simulink model "Model"  (R2024b)
settings: Solver=VariableStepAuto  StartTime=0.0  StopTime=10.0  RelTol=1e-3
libraries: simulink x5
settings Model: Creator=ethansilver  LastModifiedBy=ethansilver

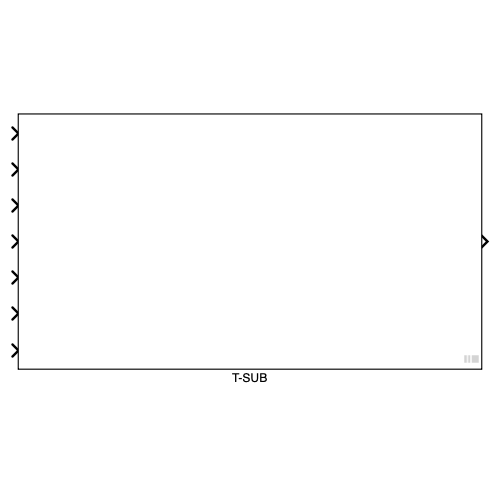
[thumbnail: Simulink's stored preview of the top-level diagram]
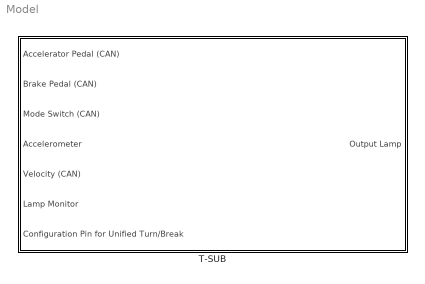
== system Model ==
  T-SUB : Subsystem

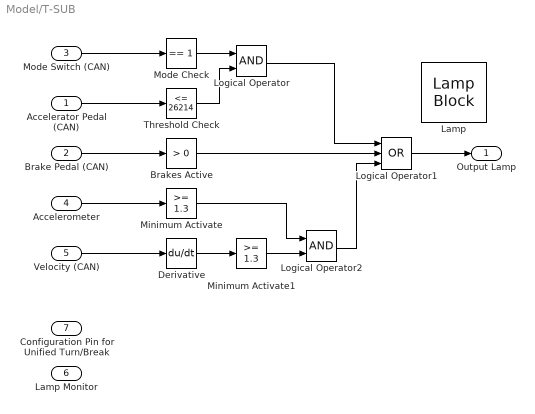
== system Model/T-SUB ==
  Accelerator Pedal (CAN) : Inport  OutMin=0  OutMax=65535  OutDataTypeStr=uint16
  Brake Pedal (CAN) : Inport  Port=2  OutMin=0  OutMax=65535  OutDataTypeStr=uint16
  Mode Switch (CAN) : Inport  Port=3  OutMin=0  OutMax=1  OutDataTypeStr=boolean
  Accelerometer : Inport  Port=4  OutMin=0  OutMax=200  OutDataTypeStr=double  Unit=m/s
  Velocity (CAN) : Inport  Port=5  OutMin=0  OutMax=200  OutDataTypeStr=double  Unit=m/s
  Lamp Monitor : Inport  Port=6  OutMin=0  OutMax=1  OutDataTypeStr=boolean
  Configuration Pin for Unified Turn/Break : Inport  Port=7  OutMin=0  OutMax=255  OutDataTypeStr=double
  Brakes Active : simulink/Logic and Bit Operations/Compare To Constant  relop=>  const=0  OutDataTypeStr=boolean
  Derivative : Derivative
  Lamp : LampBlock  LabelPosition=Hide
  Logical Operator : Logic  AllPortsSameDT=off  OutDataTypeStr=boolean
  Logical Operator1 : Logic  Operator=OR  Inputs=3  AllPortsSameDT=off  OutDataTypeStr=boolean
  Logical Operator2 : Logic  AllPortsSameDT=off  OutDataTypeStr=boolean
  Minimum Activate : simulink/Logic and Bit Operations/Compare To Constant  relop=>=  const=1.3  OutDataTypeStr=boolean
  Minimum Activate1 : simulink/Logic and Bit Operations/Compare To Constant  relop=>=  const=1.3  OutDataTypeStr=boolean
  Mode Check : simulink/Logic and Bit Operations/Compare To Constant  relop===  const=1  OutDataTypeStr=boolean
  Threshold Check : simulink/Logic and Bit Operations/Compare To Constant  relop=<=  const=26214  OutDataTypeStr=boolean
  Output Lamp : Outport
  wires:
  Accelerometer/1 -> Minimum Activate/1
  Mode Switch (CAN)/1 -> Mode Check/1
  Mode Check/1 -> Logical Operator/1
  Brake Pedal (CAN)/1 -> Brakes Active/1
  Accelerator Pedal (CAN)/1 -> Threshold Check/1
  Threshold Check/1 -> Logical Operator/2
  Logical Operator1/1 -> Output Lamp/1
  Brakes Active/1 -> Logical Operator1/2
  Logical Operator/1 -> Logical Operator1/1
  Velocity (CAN)/1 -> Derivative/1
  Derivative/1 -> Minimum Activate1/1
  Minimum Activate1/1 -> Logical Operator2/2
  Minimum Activate/1 -> Logical Operator2/1
  Logical Operator2/1 -> Logical Operator1/3
